simulink model "cdip_least_square_MN_sim"  (R2013a)
settings: Solver=ode1  StartTime=0.0  StopTime=max(t)  FixedStep=0.001  RelTol=1e-3
values from neighbouring files (symbols this model uses):
  g = 9.81e+000    (= 9.81)    [p1c321_cdip_id_pend.m]    (also in p1c322_cdip_id_least_square.m; p1c322_cdip_plot_MN.m; p1c332_adip_id_least_square.m; p1c332_adip_id_pend.m)
  lp = 2.30e-001    (= 0.23)    [p1c321_cdip_id_pend.m]    (also in p1c322_cdip_id_least_square.m; p1c322_cdip_plot_MN.m)
  mp = 1.07e-001    (= 0.107)    [p1c321_cdip_id_pend.m]    (also in p1c322_cdip_id_least_square.m; p1c322_cdip_plot_MN.m)
  Tf1 = 0.075    [p1c322_cdip_id_least_square.m]    (also in p1c322_cdip_plot_MN.m = 0.05; p1c332_adip_id_least_square.m)
  Tf2 = 0.075    [p1c322_cdip_id_least_square.m]    (also in p1c322_cdip_plot_MN.m = 0.05; p1c332_adip_id_least_square.m)
libraries: cstblocks x6
settings Model: Creator=kawata  LastModifiedBy=kawata
settings DataIOCC: SignalLoggingSaveFormat=ModelDataLogs
settings OptimizationCC: ExpressionDepthLimit=2147483647
settings DebuggingCC: FcnCallInpInsideContextMsg=UseLocalSettings
settings GRTTargetCC: CombineOutputUpdateFcns=off  GRTInterface=on

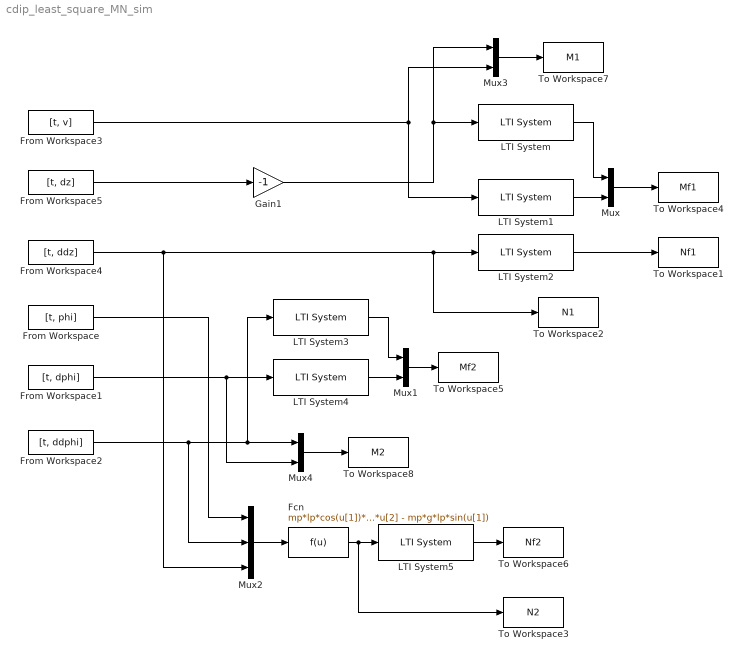
== system cdip_least_square_MN_sim ==
  Fcn : Fcn  Expr=mp*lp*cos(u[1])*u[3] - mp*lp^2*u[2] - mp*g*lp*sin(u[1])
  From Workspace : FromWorkspace  VariableName=[t, phi]  SampleTime=0
  From Workspace1 : FromWorkspace  VariableName=[t, dphi]  SampleTime=0
  From Workspace2 : FromWorkspace  VariableName=[t, ddphi]  SampleTime=0
  From Workspace3 : FromWorkspace  VariableName=[t, v]  SampleTime=0
  From Workspace4 : FromWorkspace  VariableName=[t, ddz]  SampleTime=0
  From Workspace5 : FromWorkspace  VariableName=[t, dz]  SampleTime=0
  Gain1 : Gain  Gain=-1  SaturateOnIntegerOverflow=on  OutDataTypeStr=Inherit: Same as input  ParamDataTypeStr=Inherit: Same as input
  LTI System : cstblocks/LTI System  sys=tf(1,[Tf1 1])^3  IC=[]
  LTI System1 : cstblocks/LTI System  sys=tf(1,[Tf1 1])^3  IC=[]
  LTI System2 : cstblocks/LTI System  sys=tf(1,[Tf1 1])^3  IC=[]
  LTI System3 : cstblocks/LTI System  sys=tf(1,[Tf2 1])^3  IC=[]
  LTI System4 : cstblocks/LTI System  sys=tf(1,[Tf2 1])^3  IC=[]
  LTI System5 : cstblocks/LTI System  sys=tf(1,[Tf2 1])^3  IC=[]
  Mux{,1,3..4} (4 alike) : Mux  Inputs=2
  Mux2 : Mux  Inputs=3
  To Workspace1 : ToWorkspace  VariableName=Nf1  SampleTime=-1
  To Workspace2 : ToWorkspace  VariableName=N1  SampleTime=-1
  To Workspace3 : ToWorkspace  VariableName=N2  SampleTime=-1
  To Workspace4 : ToWorkspace  VariableName=Mf1  SampleTime=-1
  To Workspace5 : ToWorkspace  VariableName=Mf2  SampleTime=-1
  To Workspace6 : ToWorkspace  VariableName=Nf2  SampleTime=-1
  To Workspace7 : ToWorkspace  VariableName=M1  SampleTime=-1
  To Workspace8 : ToWorkspace  VariableName=M2  SampleTime=-1
  wires:
  Mux1/1 -> To Workspace5/1
  LTI System3/1 -> Mux1/1
  LTI System4/1 -> Mux1/2
  From Workspace2/1 -> Mux2/2, Mux4/1, LTI System3/1
  From Workspace1/1 -> Mux4/2, LTI System4/1
  Mux2/1 -> Fcn/1
  Fcn/1 -> LTI System5/1, To Workspace3/1
  LTI System5/1 -> To Workspace6/1
  From Workspace/1 -> Mux2/1
  From Workspace4/1 -> Mux2/3, LTI System2/1, To Workspace2/1
  Mux/1 -> To Workspace4/1
  LTI System/1 -> Mux/1
  LTI System1/1 -> Mux/2
  LTI System2/1 -> To Workspace1/1
  From Workspace5/1 -> Gain1/1
  Gain1/1 -> Mux3/1, LTI System/1
  From Workspace3/1 -> Mux3/2, LTI System1/1
  Mux3/1 -> To Workspace7/1
  Mux4/1 -> To Workspace8/1
